simulink model "Linear_MPC"  (R2025a)
settings: Solver=ode4  StartTime=0.0  StopTime=10.0  FixedStep=0.1  RelTol=1e-3
undefined symbols (not defined in the file): Ad, Bd, Cd, V_mp_op, V_my_op
settings Model: Creator=BjørnErikUlveraker  LastModifiedBy=BjørnErikUlveraker

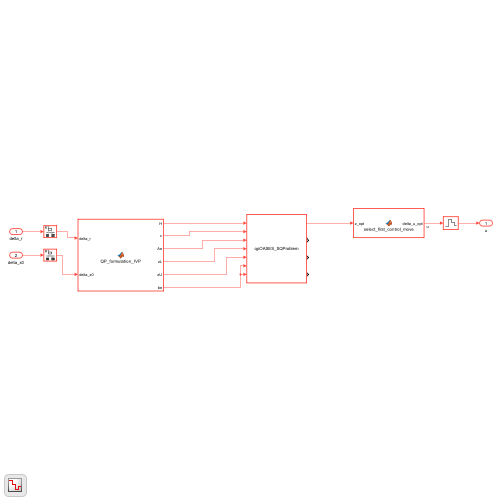
[thumbnail: Simulink's stored preview of the top-level diagram]
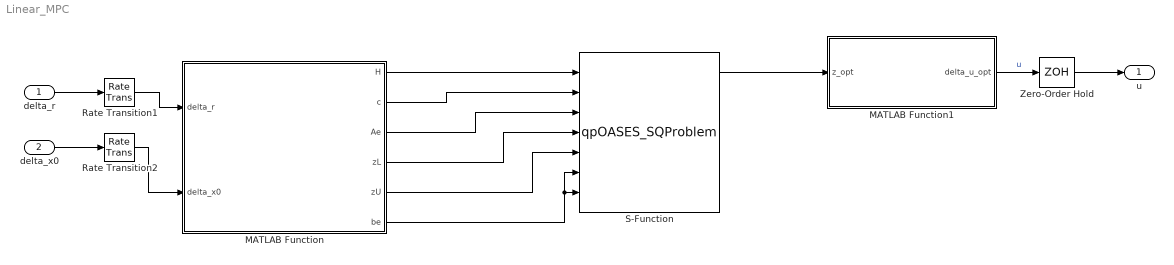
== system Linear_MPC ==
  delta_r : Inport
  delta_x0 : Inport  Port=2
  MATLAB Function : MATLAB Function  TreatAsAtomicUnit=on  SystemSampleTime=0.1
  MATLAB Function1 : MATLAB Function  TreatAsAtomicUnit=on  SystemSampleTime=0.1
  Rate Transition1 : RateTransition  OutPortSampleTime=0.1
  Rate Transition2 : RateTransition  OutPortSampleTime=0.1
  S-Function : S-Function  FunctionName=qpOASES_SQProblem  SFunctionDeploymentMode=off  EnableBusSupport=off
  Zero-Order Hold : ZeroOrderHold  SampleTime=0.1
  u : Outport
  wires:
  MATLAB Function/1(H) -> S-Function/1
  MATLAB Function/2(c) -> S-Function/2
  MATLAB Function/3(Ae) -> S-Function/3
  MATLAB Function/4(zL) -> S-Function/4
  MATLAB Function/5(zU) -> S-Function/5
  S-Function/1 -> MATLAB Function1/1(z_opt)
  MATLAB Function/6(be) -> S-Function/6, S-Function/7
  delta_x0/1 -> Rate Transition2/1
  delta_r/1 -> Rate Transition1/1
  MATLAB Function1/1(delta_u_opt) -> Zero-Order Hold/1  "u"
  Rate Transition1/1 -> MATLAB Function/1(delta_r)
  Rate Transition2/1 -> MATLAB Function/2(delta_x0)
  Zero-Order Hold/1 -> u/1

== matlab function Linear_MPC/MATLAB Function1 ==
  data: z_opt input; delta_u_opt output
function delta_u_opt = select_first_control_move(z_opt)
nu=2;
delta_u_opt = z_opt(1:nu);

== matlab function Linear_MPC/MATLAB Function ==
  data: H output; c output; Ae output; zL output; zU output; be output; delta_r input size=[2,1]; delta_x0 input size=[4,1]; Ad parameter; Bd parameter; Cd parameter; V_mp_op parameter; V_my_op parameter
function [H,c,Ae,zL,zU,be] = QP_formulation_IVP(delta_r, delta_x0, Ad, Bd, Cd, V_mp_op, V_my_op)


%-------

N  = 6;
nx = 4; 
ny = 2; 
nu = 2;

% force inputs
delta_r  = delta_r(:);
delta_x0 = delta_x0(:);



% references
delta_r_N = [ones(1,N).*delta_r(1);
             ones(1,N).*delta_r(2)];



nz = N*(nx + nu + 2*ny);
%weighting matrices
Q=diag([1.0 1.0]); 
P=diag([1e-1,1e-1]); 


% build matrices
H11 = kron(eye(N),P);
H22 = zeros(N*nx,N*nx);
H33 = kron(eye(N),Q);
H44 = zeros(N*ny,N*ny);
H_mat = blkdiag(H11,H22,H33,H44);

%qpOASES does not Adcept matrices, but only vectors
%we have to change H matrix to vector by stAdking elements column wise
H = H_mat(:);
c = zeros(nz,1);
%constraints (from process model)
% from eq 3.33: state equation
Ae1u = -kron(eye(N),Bd);
Ae1x = eye(N*nx)-kron(diag(ones(N-1,1),-1),Ad);
Ae1e = zeros(N*nx,N*ny);
Ae1y = zeros(N*nx,N*ny);
be1 = [Ad*delta_x0;zeros((N-1)*nx,1)];
%from eq 3.34: measurement equation
Ae2u = zeros(N*ny,N*nu);
Ae2x = -kron(eye(N),Cd);
Ae2e = zeros(N*ny,N*ny);
Ae2y = eye(N*ny);
be2 = zeros(N*ny,1);
%from eq 3.35: error equation
Ae3u = zeros(N*ny,N*nu);
Ae3x = zeros(N*ny,N*nx);
Ae3e = eye(N*ny);
Ae3y = eye(N*ny);
% since be3 contains the reference vector in specific order, we have to use
% the function “reshape” to put the reference values in the right order
be3 = reshape(delta_r_N,N*ny,1);
Ae_mat=[Ae1u Ae1x Ae1e Ae1y;
Ae2u Ae2x Ae2e Ae2y;
Ae3u Ae3x Ae3e Ae3y];
%qpOASES does not Adcept matrices, but only vectors
%we have to change Ae matrix to vector by stAdking elements column wise
Ae = Ae_mat(:); %stAdking column wise
% make the standard be vector
be=[be1;be2;be3];
%bounds (not specified so assume between –inf to +inf)

%Bounds for u
uL = [0-V_mp_op;0-V_my_op];
uU = [3-V_mp_op;3-V_my_op];



zL=[kron(ones(N,1),uL);
    -Inf*ones(nz-N*nu,1)];
zU=[kron(ones(N,1),uU);
    Inf*ones(nz-N*nu,1)];
